simulink model "rectifier_reminder"  (R2020b)
settings: Solver=VariableStepAuto  StartTime=0.0  StopTime=0.3  RelTol=1e-3
model workspace (MAT data in the model file):
  Ln = 0.008
  Rn = 0.01
  Tdiscrete = 2e-06
  Tpwm_r = 0.0005
  Udref = 1600
  Un = 1000
libraries: powerlib x16, pid_lib x1, simulink x1, eeSinusoidalMeasurementV2 x1
settings Model: Creator=messer  LastModifiedBy=messer
settings SolverCC: ZeroCrossAlgorithm=Adaptive
settings DebuggingCC: IgnoredZcDiagnostic=none

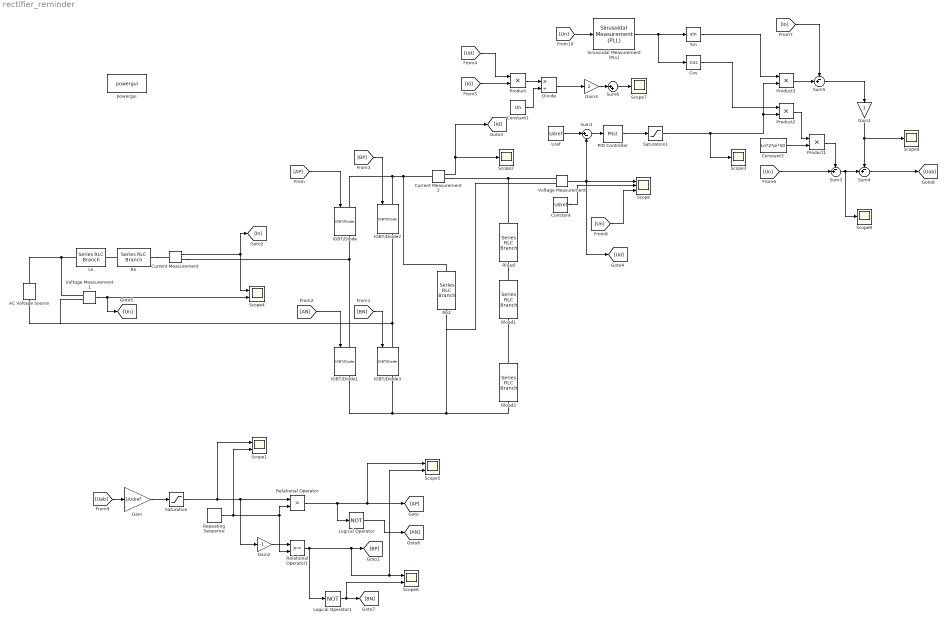
== system rectifier_reminder ==
  AC Voltage Source : powerlib/Electrical Sources/AC Voltage Source  Amplitude=Un  Phase=0  Frequency=50  SampleTime=0  Measurements=None  BusType=swing  Pref=10e3  Qref=0  Qmin=-inf  Qmax=+inf
  Constant : Constant  Value=Udref
  Constant1 : Constant  Value=Un
  Constant3 : Constant  Value=Ln*2*pi*50
  Cos : Trigonometry  Operator=cos
  Current Measurement : powerlib/Measurements/Current Measurement  PhasorSimulation=off  OutputType=Complex  PSBequivalent=0
  Current Measurement2 : powerlib/Measurements/Current Measurement  PhasorSimulation=off  OutputType=Complex  PSBequivalent=0
  Divide : Product  Inputs=*/
  Gain : Gain  Gain=1/Udref
  Gain1 : Gain
  Gain2 : Gain  Gain=-1
  Gain3 : Gain  Gain=2
  IGBT/Diode{,1..3} (4 alike) : powerlib/Power Electronics/IGBT//Diode  Ron=1e-3  Rs=1e5  Cs=inf  Measurements=on
  Ln : powerlib/Elements/Series RLC Branch  LConnTagsString=__new0  RConnTagsString=__new0  BranchType=L  Resistance=1  Inductance=Ln  SetiL0=off  InitialCurrent=0  Capacitance=1e-6  Setx0=off  InitialVoltage=0  Measurements=None
  Logical Operator : Logic  Operator=NOT  AllPortsSameDT=off  OutDataTypeStr=boolean
  Logical Operator1 : Logic  Operator=NOT  AllPortsSameDT=off  OutDataTypeStr=boolean
  PID Controller : pid_lib/PID Controller  Controller=PI  Form=Parallel  TimeDomain=Continuous-time  UseExternalTs=off  SampleTime=-1  IntegratorMethod=Forward Euler  FilterMethod=Forward Euler  ControllerParametersSource=internal  P=1.3  I=2.5  D=0  UseFilter=on  N=100  TunerSelectOption=Transfer Function Based (PID Tuner App)  InitialConditionSource=internal  InitialConditionForIntegrator=0  InitialConditionForFilter=0  DifferentiatorICPrevScaledInput=0  ExternalReset=none  TrackingMode=off  Kt=1  LimitOutput=off  SatLimitsSource=internal  UpperSaturationLimit=inf  LowerSaturationLimit=-inf  LinearizeAsGain=on  AntiWindupMode=none  Kb=1  POutMin=[]  POutMax=[]  IOutMin=[]  IOutMax=[]  DOutMin=[]  DOutMax=[]  NOutMin=[]  NOutMax=[]  SumOutMin=[]  SumOutMax=[]  SaturationOutMin=[]  SaturationOutMax=[]  PParamMin=[]  PParamMax=[]  IParamMin=[]  IParamMax=[]  DParamMin=[]  DParamMax=[]  NParamMin=[]  NParamMax=[]  KbParamMin=[]  KbParamMax=[]  KtParamMin=[]  KtParamMax=[]  KbOutMin=[]  KbOutMax=[]  KtOutMin=[]  KtOutMax=[]  IntegratorOutMin=[]  IntegratorOutMax=[]  FilterOutMin=[]  FilterOutMax=[]  SumI1OutMin=[]  SumI1OutMax=[]  SumI2OutMin=[]  SumI2OutMax=[]  SumI3OutMin=[]  SumI3OutMax=[]  SumI4OutMin=[]  SumI4OutMax=[]  SumDOutMin=[]  SumDOutMax=[]  DifferentiatorOutMin=[]  DifferentiatorOutMax=[]  FilterDiffOutCoefMin=[]  FilterDiffOutCoefMax=[]  ReciprocalOutMin=[]  ReciprocalOutMax=[]  SumDenOutMin=[]  SumDenOutMax=[]  SumNumOutMin=[]  SumNumOutMax=[]  DivideOutMin=[]  DivideOutMax=[]  UdiffTsProdOutMin=[]  UdiffTsProdOutMax=[]  NTsProdOutMin=[]  NTsProdOutMax=[]  UintegralTsProdOutMin=[]  UintegralTsProdOutMax=[]  UngainTsProdOutMin=[]  UngainTsProdOutMax=[]  IntegratorContinuousStateAttributes=''  IntegratorStateMustResolveToSignalObject=off  IntegratorRTWStateStorageClass=Auto  FilterContinuousStateAttributes=''  FilterStateMustResolveToSignalObject=off  FilterRTWStateStorageClass=Auto  ParallelPVariant=InternalParameters  IdealPVariant=Disabled  IVariant=InternalParameters  DVariant=Disabled  IntegratorVariant=Continuous  SatVariant=Disabled  AWVariant=Passthrough  PCopyVariant=Disabled  TRVariant=Disabled  FdbkBlocksVariant=Forward  IdealPFdbkVariant=Disabled  SatFdbkVariant=Disabled  DerivativeFilterVariant=Disabled  NVariant=Disabled  NCopyVariant=Disabled_SignalSpec  FilterICVariant=Disabled  IntegratorICVariant=InternalICs  ExternalResetVariant=Disabled  TRSumVariant=Passthrough  SumFdbkVariant=Disabled  SumVariant=Sum_PI  TsampFilterVariant=InternalTs  TsampNgainVariant=Passthrough  TsampIntegralVariant=Passthrough  ExternalSaturationOutDataTypeStr=Inherit: Same as second input
  Product{,1..3} (4 alike) : Product
  Relational Operator : RelationalOperator  Operator=>  OutDataTypeStr=boolean  RndMeth=Simplest
  Relational Operator1 : RelationalOperator  OutDataTypeStr=boolean  RndMeth=Simplest
  Repeating Sequence : simulink/Sources/Repeating Sequence  rep_seq_t=[0 Tpwm_r/2 Tpwm_r]  rep_seq_y=[-1 1 -1]
  Rload : powerlib/Elements/Series RLC Branch  LConnTagsString=__new0  RConnTagsString=__new0  BranchType=R  Resistance=300  Inductance=1e-3  SetiL0=off  InitialCurrent=0  Capacitance=1e-6  Setx0=off  InitialVoltage=0  Measurements=None
  Rload1 : powerlib/Elements/Series RLC Branch  LConnTagsString=__new0  RConnTagsString=__new0  BranchType=R  Resistance=1  Inductance=1e-3  SetiL0=off  InitialCurrent=0  Capacitance=1e-6  Setx0=off  InitialVoltage=0  Measurements=None
  Rload2 : powerlib/Elements/Series RLC Branch  LConnTagsString=__new0  RConnTagsString=__new0  BranchType=R  Resistance=1  Inductance=1e-3  SetiL0=off  InitialCurrent=0  Capacitance=1e-6  Setx0=off  InitialVoltage=0  Measurements=None
  Rn : powerlib/Elements/Series RLC Branch  LConnTagsString=__new0  RConnTagsString=__new0  BranchType=R  Resistance=Rn  Inductance=1e-3  SetiL0=off  InitialCurrent=0  Capacitance=1e-6  Setx0=off  InitialVoltage=0  Measurements=None
  Rn2 : powerlib/Elements/Series RLC Branch  LConnTagsString=__new0  RConnTagsString=__new0  BranchType=C  Resistance=0.05  Inductance=1e-3  SetiL0=off  InitialCurrent=0  Capacitance=5e-3  Setx0=off  InitialVoltage=0  Measurements=None
  Saturation : Saturate  UpperLimit=1  LowerLimit=-1
  Saturation1 : Saturate  UpperLimit=1000  LowerLimit=-1000
  Scope : Scope  NumInputPorts=3
  Scope{1,4..6} (4 alike) : Scope  NumInputPorts=2
  Scope{2..3,7..9} (5 alike) : Scope
  Sin : Trigonometry
  Sinusoidal Measurement (PLL) : eeSinusoidalMeasurementV2/Sinusoidal Measurement (PLL)  Ki_PD=1000  Kp_LF=400  Ki_LF=20000  F0=60  Theta0=0  Mag0=1  Ts=-1
      settings: SourceProductBaseCode=PS
  Sum1 : Sum  Inputs=|+-
  Sum3 : Sum  Inputs=-+|
  Sum4 : Sum  Inputs=-+|
  Sum5 : Sum  Inputs=-+|
  Sum6 : Sum  Inputs=|++
  Uref : Constant  Value=Udref
  Voltage Measurement : powerlib/Measurements/Voltage Measurement  PhasorSimulation=off  OutputType=Complex  PSBequivalent=0
  Voltage Measurement1 : powerlib/Measurements/Voltage Measurement  PhasorSimulation=off  OutputType=Complex  PSBequivalent=0
  powergui : powerlib/powergui  Priority=1  SimulationMode=Discrete  SampleTime=1e-6  frequency=60  Iterations=50  frequencyindice=50  Pbase=100e6  ErrMax=1e-4  UnitsV=kV  UnitsW=MW  buscounter=0  FunctionMessages=off  echomessages=off  EnableUseOfTLC=off  CurrentSourceSwitches=off  DisableSnubberDevices=off  DisableRonSwitches=off  DisableVfSwitches=off  DisplayEquations=off  AutomaticDiscreteSolvers=off  SolverType=Tustin/Backward Euler (TBE)  Interpol=off  ExternalGateDelay=off  methode=off  Ts=100  x0status=blocks  SPID=on  SwTol=0  HookPort=off  NonlinearTolerance=1e-4  nMaxIteration=100  ContinueOnMaxIteration=off  RestoreLinks=warning  ResistiveCurrentMeasurement=off  Frange=[0:2:500]  Ylog=off  Xlog=on  ShowGrid=off  save=off  variable=ZData  structure=0  ZoomFFT=off  StartTime=0.0  cycles=1  DisplayStyle=1  fundamental=60  FreqAxis=off  MaxFrequency=1000  frequencyindicesteady=1  RmsSteady=1  display=off
  wires:
  Voltage Measurement/1 -> Sum1/2, Scope/1, [Ud]
  Current Measurement/1 -> [In], Scope4/1
  Uref/1 -> Sum1/1
  Sum1/1 -> PID Controller/1
  Current Measurement2/1 -> [Id], Scope2/1
  [Id] -> Product/2
  [Ud] -> Product/1
  Voltage Measurement1/1 -> Scope4/2, [Un]
  PID Controller/1 -> Saturation1/1
  Constant3/1 -> Product1/2
  Cos/1 -> Product2/1
  [Un] -> Sum3/2
  Sum3/1 -> Scope8/1, Sum4/2
  Sin/1 -> Product3/1
  Product3/1 -> Sum5/2
  [In] -> Sum5/1
  Sum5/1 -> Gain1/1
  Product2/1 -> Product1/1
  Product1/1 -> Sum3/1
  [AP] -> IGBT/Diode/1
  [AN] -> IGBT/Diode1/1
  [BP] -> IGBT/Diode2/1
  [BN] -> IGBT/Diode3/1
  Product/1 -> Divide/1
  Constant1/1 -> Divide/2
  Divide/1 -> Gain3/1
  Sum6/1 -> Scope7/1
  Constant/1 -> Scope/2
  Gain3/1 -> Sum6/1
  [Un] -> Scope/3
  Gain/1 -> Saturation/1
  Gain2/1 -> Relational Operator1/1
  Logical Operator1/1 -> Scope6/2, [BN]
  Relational Operator/1 -> Logical Operator/1, Scope5/1, [AP]
  Relational Operator1/1 -> Logical Operator1/1, Scope5/2, Scope6/1, [BP]
  Logical Operator/1 -> [AN]
  [Uab] -> Gain/1
  Repeating Sequence/1 -> Scope1/2, Relational Operator1/2, Relational Operator/2
  Sum4/1 -> [Uab]
  [Un] -> Sinusoidal Measurement (PLL)/1
  Sinusoidal Measurement (PLL)/2 -> Cos/1, Sin/1
  Gain1/1 -> Sum4/1, Scope9/1
  Saturation/1 -> Scope1/1, Gain2/1, Relational Operator/1
  Saturation1/1 -> Product2/2, Product3/2, Scope3/1
  connections:
  Rn/LConn1 -- Ln/RConn1
  Ln/LConn1 -- Voltage Measurement1/LConn1 -- AC Voltage Source/RConn1
  IGBT/Diode1/LConn1 -- IGBT/Diode/RConn1 -- Current Measurement/RConn1
  IGBT/Diode3/LConn1 -- Voltage Measurement1/LConn2 -- AC Voltage Source/LConn1 -- IGBT/Diode2/RConn1
  IGBT/Diode1/RConn1 -- IGBT/Diode3/RConn1 -- Voltage Measurement/LConn2 -- Rn2/RConn1 -- Rload2/RConn1
  Rn/RConn1 -- Current Measurement/LConn1
  Current Measurement2/LConn1 -- IGBT/Diode2/LConn1 -- IGBT/Diode/LConn1 -- Rn2/LConn1
  Rload1/RConn1 -- Rload2/LConn1
  Rload/RConn1 -- Rload1/LConn1
  Voltage Measurement/LConn1 -- Current Measurement2/RConn1 -- Rload/LConn1
